simulink model "vehicle"  (R2018a)
settings: Solver=FixedStepAuto  StartTime=0.0  StopTime=100  RelTol=1e-3  EnableMultiTasking=on
libraries: fuzblock x1
settings Model: Creator=Lenovo  LastModifiedBy=Kasra
settings DataIOCC: LimitDataPoints=on
settings OptimizationCC: LifeSpan=inf
settings DebuggingCC: MaxConsecutiveZCsMsg=none  AllowSymbolicDim=off  SFUnexpectedBacktrackingDiag=warning  SFNoUnconditionalDefaultTransitionDiag=warning  SFExecutionAtInitializationDiag=none
settings ModelReferenceCC: PropagateSignalLabelsOutOfModel=off
settings CodeAppCC: StateflowObjectComments=on
settings GRTTargetCC: TargetLangStandard=C89/C90 (ANSI)
settings ConfigComp: CovMetricSettings=dw  CovHtmlReporting=on  CovSaveCumulativeToWorkspaceVar=on  CovSaveSingleToWorkspaceVar=on  CovExternalEMLEnable=off

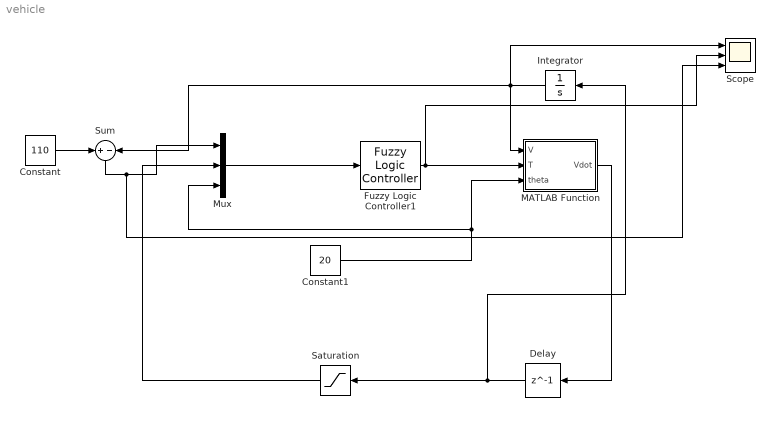
== system vehicle ==
  Constant : Constant  Value=110
  Constant1 : Constant  Value=20
  Delay : Delay  DelayLength=1
  Fuzzy Logic Controller1 : fuzblock/Fuzzy Logic  Controller  FIS='controller2'  OutputSampleNumber=101  DataType=double  FuzzifiedInputs=off  RuleFiringStrengths=off  RuleOutputs=off  AggregatedOutputs=off  SimulateUsing=Interpreted execution  OutOfRangeInputValueMessage=warning  NoRuleFiredMessage=warning  EmptyOutputFuzzySetMessage=warning
  Integrator : Integrator
  MATLAB Function : MATLAB Function  TreatAsAtomicUnit=on
  Mux : Mux  Inputs=3
  Saturation : Saturate
  Scope : Scope  NumInputPorts=3
  Sum : Sum  Inputs=+-
  wires:
  Constant/1 -> Sum/1
  Mux/1 -> Fuzzy Logic Controller1/1
  Sum/1 -> Scope/3, Mux/1
  Constant1/1 -> MATLAB Function/3(theta), Mux/3
  Integrator/1 -> Scope/1, MATLAB Function/1(V), Sum/2
  Saturation/1 -> Mux/2
  Fuzzy Logic Controller1/1 -> MATLAB Function/2(T), Scope/2
  Delay/1 -> Saturation/1, Integrator/1
  MATLAB Function/1(Vdot) -> Delay/1

== matlab function vehicle/MATLAB Function ==
  data: V input; Vdot output; T input; theta input
function Vdot = vehichle(V, T , theta)

Vdot = -0.1*V + T -0.1*theta;
